simulink library "MeldasLibrary"  (R2016b)
settings: Solver=VariableStepAuto  StartTime=0.0  StopTime=10.0  RelTol=1e-3
libraries: simulink x2
settings Model: Creator=mulusoy  LastModifiedBy=mulusoy
settings DebuggingCC: SFUnconditionalPathOutOfParentDiag=warning  SFUnreachableStateOrJunctionDiag=warning  SFDanglingTransitionDiag=warning
settings CodeAppCC: CustomSymbolStrSimulinkFcn=$N
settings ConfigComp: CovMetricSettings=dswe

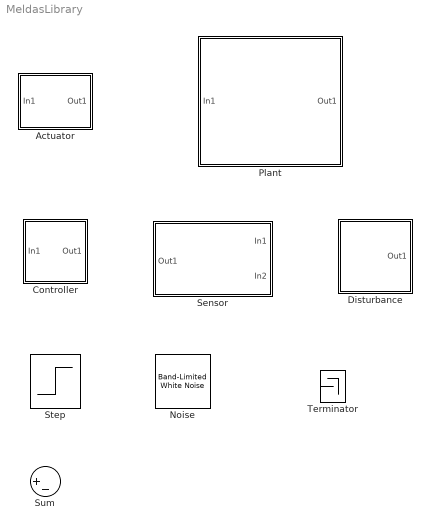
== system MeldasLibrary ==
  Actuator : Subsystem
      mask Display: image('.\Mask icons\Foot on pedal.png');
  Controller : Subsystem
      mask Display: image('.\Mask icons\Brain.jpg');
  Disturbance : Subsystem
      mask Display: image('.\Mask icons\Hill.jpg')
  Noise : simulink/Sources/Band-Limited White Noise  Cov=[0.01]  Ts=0.1  seed=[23341]
  Plant : Subsystem  Variant=on  mask{passengerNumber=Driver only}
      mask prompts: passengerNumber "Select Vehicle Type"
      mask TypeOptions passengerNumber: Driver only | Passengers | Passengers and elephant
      mask Callback passengerNumber:
      | % Get the selected passenger number
      | passengerNumberStr = get_param(gcbh, 'passengerNumber');
      | 
      | % Set the active variant
      | if strcmpi(passengerNumberStr, 'Driver only')
      |     evalin('base','passengerNumber = 1;');
      | elseif strcmpi(passengerNumberStr, 'Passengers')
      |     evalin('base','passengerNumber = 2;');
      | else
      |     evalin('base','passengerNumber = 3;');
      | end
      mask Display:
      | % Update the icon based on the value of passengerNumber
      | if passengerNumber == 1
      |    image('.\Mask icons\Car.jpg');
      | elseif passengerNumber == 2
      |    image('.\Mask icons\Car with passengers.jpg');
      | else
      |    image('.\Mask icons\Car with elephant.jpg');
      | end
  Sensor : Subsystem
      mask Display: image('.\Mask icons\Monitoring speed.jpg');
  Step : Step  After=20  SampleTime=0
  Sum : Sum  Inputs=|+-
  Terminator : Terminator

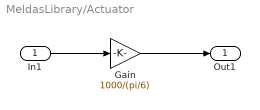
== system MeldasLibrary/Actuator ==
  In1 : Inport
  Gain : Gain  Gain=1000/(pi/6)
  Out1 : Outport
  wires:
  In1/1 -> Gain/1
  Gain/1 -> Out1/1

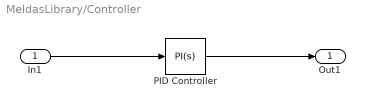
== system MeldasLibrary/Controller ==
  In1 : Inport
  PID Controller : simulink/Continuous/PID Controller  Controller=PI  TimeDomain=Continuous-time  SampleTime=-1  IntegratorMethod=Forward Euler  FilterMethod=Forward Euler  Form=Parallel  UseFilter=on  ControllerParametersSource=internal  P=0.0294195707767973  I=0.00147097853883986  D=0  N=100  InitialConditionSource=internal  InitialConditionForIntegrator=0  InitialConditionForFilter=0  ExternalReset=none  LimitOutput=off  UpperSaturationLimit=inf  LowerSaturationLimit=-inf  LinearizeAsGain=on  AntiWindupMode=none  Kb=1  TrackingMode=off  Kt=1  PParamMin=[]  PParamMax=[]  IParamMin=[]  IParamMax=[]  DParamMin=[]  DParamMax=[]  NParamMin=[]  NParamMax=[]  KbParamMin=[]  KbParamMax=[]  KtParamMin=[]  KtParamMax=[]  POutMin=[]  POutMax=[]  IOutMin=[]  IOutMax=[]  DOutMin=[]  DOutMax=[]  NOutMin=[]  NOutMax=[]  KbOutMin=[]  KbOutMax=[]  KtOutMin=[]  KtOutMax=[]  IntegratorOutMin=[]  IntegratorOutMax=[]  FilterOutMin=[]  FilterOutMax=[]  SumOutMin=[]  SumOutMax=[]  SumI1OutMin=[]  SumI1OutMax=[]  SumI2OutMin=[]  SumI2OutMax=[]  SumI3OutMin=[]  SumI3OutMax=[]  SumDOutMin=[]  SumDOutMax=[]  SaturationOutMin=[]  SaturationOutMax=[]  IntegratorContinuousStateAttributes=''  IntegratorStateMustResolveToSignalObject=off  IntegratorRTWStateStorageClass=Auto  FilterContinuousStateAttributes=''  FilterStateMustResolveToSignalObject=off  FilterRTWStateStorageClass=Auto  DifferentiatorICPrevScaledInput=0  DifferentiatorOutMin=[]  DifferentiatorOutMax=[]
  Out1 : Outport
  wires:
  PID Controller/1 -> Out1/1
  In1/1 -> PID Controller/1

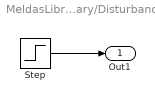
== system MeldasLibrary/Disturbance ==
  Step : Step  Time=200  After=-1000*9.81*sin(pi/45)  SampleTime=0
  Out1 : Outport
  wires:
  Step/1 -> Out1/1

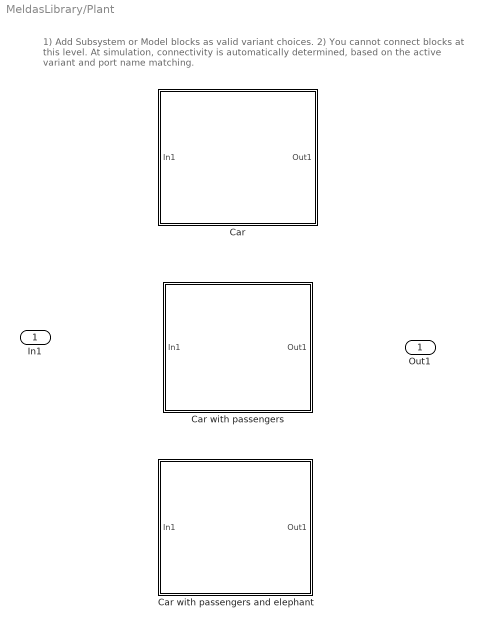
== system MeldasLibrary/Plant ==
  note: 1) Add Subsystem or Model blocks as valid variant choices.
      | 2) You cannot connect blocks at this level. At simulation, connectivity is automatically
      | determined, based on the active variant and port name matching.
  In1 : Inport
  Car : Subsystem  VariantControl=Driver
      mask Display: image('.\Mask icons\Car.jpg');
  Car with passengers : Subsystem  VariantControl=Passengers
      mask Display: image('.\Mask icons\Car with passengers.jpg');
  Car with passengers and elephant : Subsystem  VariantControl=Elephant
      mask Display: image('.\Mask icons\Car with elephant.jpg');
  Out1 : Outport

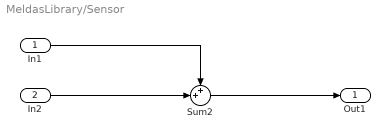
== system MeldasLibrary/Sensor ==
  In1 : Inport
  In2 : Inport  Port=2
  Sum2 : Sum  Inputs=++|
  Out1 : Outport
  wires:
  In1/1 -> Sum2/1
  In2/1 -> Sum2/2
  Sum2/1 -> Out1/1

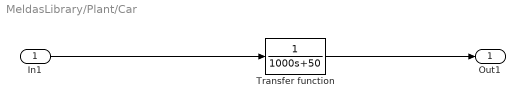
== system MeldasLibrary/Plant/Car ==
  "In1 " : Inport
  Transfer function : TransferFcn  Denominator=[1000 50]
  Out1 : Outport
  wires:
  "In1 "/1 -> Transfer function/1
  Transfer function/1 -> Out1/1

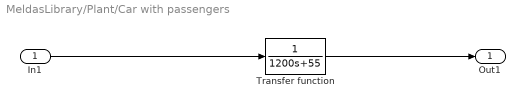
== system MeldasLibrary/Plant/Car with passengers ==
  "In1 " : Inport
  Transfer function : TransferFcn  Denominator=[1200 55]
  Out1 : Outport
  wires:
  Transfer function/1 -> Out1/1
  "In1 "/1 -> Transfer function/1

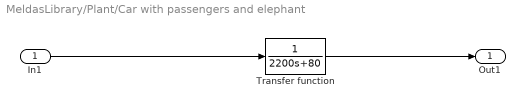
== system MeldasLibrary/Plant/Car with passengers and elephant ==
  "In1 " : Inport
  Transfer function : TransferFcn  Denominator=[2200 80]
  Out1 : Outport
  wires:
  "In1 "/1 -> Transfer function/1
  Transfer function/1 -> Out1/1
